simulink model "control"  (R2020a)
settings: Solver=FixedStepDiscrete  StartTime=0.0  StopTime=1  FixedStep=0.0005  RelTol=1e-3  EnableMultiTasking=on
undefined symbols (not defined in the file): acc_calmax1, acc_calmax2, acc_calmin1, acc_calmin2, akemancanshu, bre, bre_calmax, bre_calmin, ecucoder_acal, I_AN01_5K1, I_AN03_5V, I_AN04_5V, kd, ki, kp, leftmax, O_SW06_HS1A, rightmax, T_add, T_del, tiaoshi, zhiling
libraries: ec5744lib x252, canmsglib x92, simulink x5
(part 5 of 9)

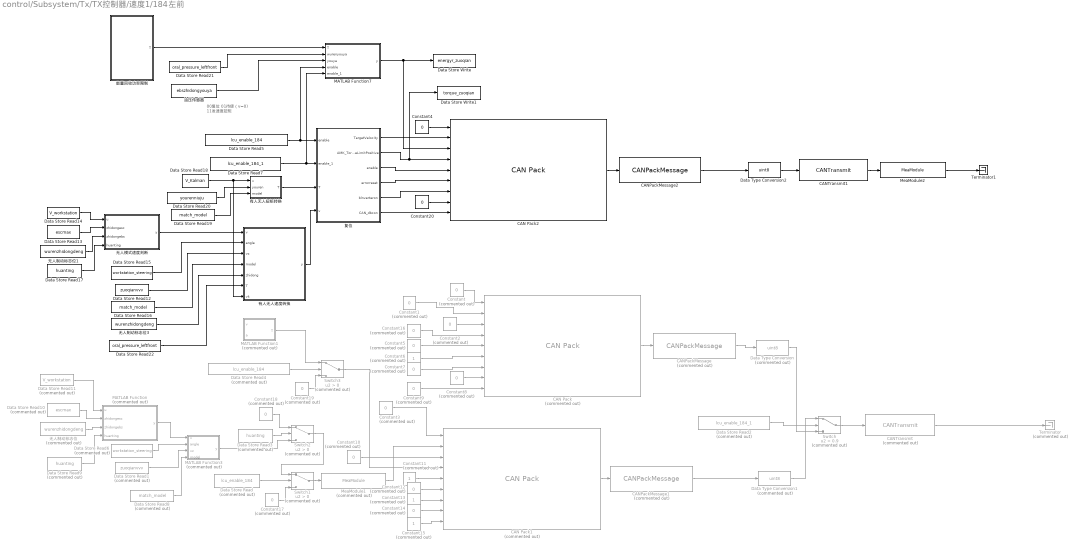
== system control/Subsystem/Tx/TX控制器/速度1/184左前 ==
  note: 00复位
      | 01待使（v=0)
      | 11发速度扭矩
  CAN Pack : canmsglib/CAN Pack  Commented=on  CANdbFile=D:\desktop\CANdbc\enable.dbc  MsgList=(none)  MsgName=first_enable  MsgIDType=Standard (11-bit identifier)  MsgIdentifier=388  MsgLength=8  Remote=off  ApplyMinMax=off  BusOutput=off  SignalInfo={'AMK_Reserve','12','4','LE','signed','Standard','0','1','0','0','15';'AMK_TargetVelocity','16','16','LE','signed','Standard','0','1','0','0','65535';'AMK_TorqueLimitNegativ','48','16','LE','signed','Standard','0','1','0','0','65535';'AMK_TorqueLimitPositiv','32','16','LE','signed','Standard','0','1','0','0','65535';'AMK_bEnable','10','1','LE','unsigned','Standard','0','1','0','0','1';'AMK_bErrorReset','11','1','LE','unsigned','Standard','0','1','0','0','1';'AMK_bInverterOn','8','1','LE','unsigned','Standard','0','1','0','0','1';'AMK_bReserve','0','8','LE','unsigned','Standard','0','1','0','0','255';'CAN_bdcon','9','1','LE','unsigned','Standard','0','1','0','0','1'}
      settings: SourceProductBaseCode=ME,XP,VN  DataFormat=CANdb specified signals
  CAN Pack1 : canmsglib/CAN Pack  Commented=on  CANdbFile=D:\desktop\CANdbc\enable.dbc  MsgList=(none)  MsgName=first_enable  MsgIDType=Standard (11-bit identifier)  MsgIdentifier=388  MsgLength=8  Remote=off  ApplyMinMax=off  BusOutput=off  SignalInfo={'AMK_Reserve','12','4','LE','signed','Standard','0','1','0','0','15';'AMK_TargetVelocity','16','16','LE','signed','Standard','0','1','0','0','65535';'AMK_TorqueLimitNegativ','48','16','LE','signed','Standard','0','1','0','0','65535';'AMK_TorqueLimitPositiv','32','16','LE','signed','Standard','0','1','0','0','65535';'AMK_bEnable','10','1','LE','unsigned','Standard','0','1','0','0','1';'AMK_bErrorReset','11','1','LE','unsigned','Standard','0','1','0','0','1';'AMK_bInverterOn','8','1','LE','unsigned','Standard','0','1','0','0','1';'AMK_bReserve','0','8','LE','unsigned','Standard','0','1','0','0','255';'CAN_bdcon','9','1','LE','unsigned','Standard','0','1','0','0','1'}
      settings: SourceProductBaseCode=ME,XP,VN  DataFormat=CANdb specified signals
  CAN Pack2 : canmsglib/CAN Pack  CANdbFile=C:\Users\86155\Desktop\HRT2024\qkx\can\enable.dbc  MsgList=first_enable  MsgName=first_enable  MsgIDType=Standard (11-bit identifier)  MsgIdentifier=388  MsgLength=8  Remote=off  ApplyMinMax=off  BusOutput=off  SignalInfo={'AMK_Reserve','12','4','LE','signed','Standard','0','1','0','-8','7';'AMK_TargetVelocity','16','16','LE','signed','Standard','0','1','0','-32768','32767';'AMK_TorqueLimitNegativ','48','16','LE','signed','Standard','0','1','0','-32768','32767';'AMK_TorqueLimitPositiv','32','16','LE','signed','Standard','0','1','0','-32768','32767';'AMK_bEnable','10','1','LE','unsigned','Standard','0','1','0','0','1';'AMK_bErrorReset','11','1','LE','unsigned','Standard','0','1','0','0','1';'AMK_bInverterOn','8','1','LE','unsigned','Standard','0','1','0','0','1';'AMK_bReserve','0','8','LE','unsigned','Standard','0','1','0','0','255';'CAN_bdcon','9','1','LE','unsigned','Standard','0','1','0','0','1'}
      settings: SourceProductBaseCode=ME,XP,VN  DataFormat=CANdb specified signals
  CANPackMessage : ec5744lib/RapidECU_U4B/04CANCommunication/CANPackMessage  Commented=on  datalength=8  sampletime=-1
      settings: SourceProductName=ECUCoder for MPC5744
  CANPackMessage1 : ec5744lib/RapidECU_U4B/04CANCommunication/CANPackMessage  Commented=on  datalength=8  sampletime=-1
      settings: SourceProductName=ECUCoder for MPC5744
  CANPackMessage2 : ec5744lib/RapidECU_U4B/04CANCommunication/CANPackMessage  datalength=8  sampletime=-1
      settings: SourceProductName=ECUCoder for MPC5744
  CANTransmit : ec5744lib/RapidECU_U4B/04CANCommunication/CANTransmit  Commented=on  canmodule=0  canbuffer=8  canmessageid=hex2dec('184')  canmessagetype=Standard(11-bit ID)  datalength=8  sampletime=-1
      settings: SourceProductName=ECUCoder for MPC5744
  CANTransmit1 : ec5744lib/RapidECU_U4B/04CANCommunication/CANTransmit  canmodule=0  canbuffer=8  canmessageid=hex2dec('184')  canmessagetype=Standard(11-bit ID)  datalength=8  sampletime=-1
      settings: SourceProductName=ECUCoder for MPC5744
  Constant{,1..3,5,7..10,12,14,16..17,19} (14 alike) : Constant  Commented=on  Value=0  SampleTime=-1
  Constant{6,11,13,15} (4 alike) : Constant  Commented=on  SampleTime=-1
  Constant18 : Constant  Commented=on  Value=0
  Constant20 : Constant  Value=0  SampleTime=-1
  Constant4 : Constant  Value=0  SampleTime=-1
  Data Store Read : DataStoreRead  Commented=on  DataStoreName=lcu_enable_184
  Data Store Read1 : DataStoreRead  Commented=on  DataStoreName=zuoqianvvv
  Data Store Read10 : DataStoreRead  Commented=on  DataStoreName=escmax
  Data Store Read11 : DataStoreRead  Commented=on  DataStoreName=V_workstation
  Data Store Read12 : DataStoreRead  DataStoreName=zuoqianvvv
  Data Store Read13 : DataStoreRead  DataStoreName=escmax
  Data Store Read14 : DataStoreRead  DataStoreName=V_workstation
  Data Store Read15 : DataStoreRead  DataStoreName=workstation_steering
  Data Store Read16 : DataStoreRead  DataStoreName=match_model
  Data Store Read17 : DataStoreRead  DataStoreName=huanting
  Data Store Read18 : DataStoreRead  DataStoreName=V_Kalman
  Data Store Read19 : DataStoreRead  DataStoreName=match_model
  Data Store Read2 : DataStoreRead  Commented=on  DataStoreName=lcu_enable_184_1
  Data Store Read20 : DataStoreRead  DataStoreName=yourenniuju
  Data Store Read21 : DataStoreRead  DataStoreName=oral_pressure_leftfront
  Data Store Read22 : DataStoreRead  DataStoreName=oral_pressure_leftfront
  Data Store Read3 : DataStoreRead  Commented=on  DataStoreName=huanting
  Data Store Read4 : DataStoreRead  Commented=on  DataStoreName=lcu_enable_184
  Data Store Read5 : DataStoreRead  DataStoreName=lcu_enable_184
  Data Store Read6 : DataStoreRead  Commented=on  DataStoreName=workstation_steering
  Data Store Read7 : DataStoreRead  DataStoreName=lcu_enable_184_1
  Data Store Read8 : DataStoreRead  Commented=on  DataStoreName=match_model
  Data Store Read9 : DataStoreRead  Commented=on  DataStoreName=huanting
  Data Store Write : DataStoreWrite  DataStoreName=energyr_zuoqian
  Data Store Write1 : DataStoreWrite  DataStoreName=torque_zuoqian
  Data Type Conversion : DataTypeConversion  Commented=on  OutDataTypeStr=uint8
  Data Type Conversion1 : DataTypeConversion  Commented=on  OutDataTypeStr=uint8
  Data Type Conversion2 : DataTypeConversion  OutDataTypeStr=uint8
  MATLAB Function : MATLAB Function  Commented=on  TreatAsAtomicUnit=on
  MATLAB Function1 : MATLAB Function  Commented=on  TreatAsAtomicUnit=on
  MATLAB Function3 : MATLAB Function  Commented=on  TreatAsAtomicUnit=on
  MATLAB Function7 : MATLAB Function  TreatAsAtomicUnit=on
  MeaModule1 : ec5744lib/RapidECU_U4B/07Calibration/MeaModule  Commented=on  signal=Vfirst
      settings: SourceProductName=ECUCoder for MPC5744
  MeaModule2 : ec5744lib/RapidECU_U4B/07Calibration/MeaModule  signal=V184
      settings: SourceProductName=ECUCoder for MPC5744
  Switch : Switch  Commented=on  Criteria=u2 > Threshold  Threshold=0.9
  Switch1 : Switch  Commented=on  Criteria=u2 > Threshold
  Switch2 : Switch  Commented=on  Criteria=u2 > Threshold
  Switch3 : Switch  Commented=on  Criteria=u2 > Threshold
  Terminator : Terminator  Commented=on
  Terminator1 : Terminator
  复位 : MATLAB Function  TreatAsAtomicUnit=on
  无人制动标志位 : DataStoreRead  Commented=on  DataStoreName=wurenzhidongdeng
  无人制动标志位1 : DataStoreRead  DataStoreName=wurenzhidongdeng
  无人制动标志位3 : DataStoreRead  DataStoreName=wurenzhidongdeng
  无人模式速度判断 : MATLAB Function  TreatAsAtomicUnit=on
  有人无人扭矩转换 : MATLAB Function  TreatAsAtomicUnit=on
  有人无人速度转换 : MATLAB Function  TreatAsAtomicUnit=on
  油压传感器 : DataStoreRead  DataStoreName=ebszhidongyouya
  能量回收功率限制 : Subsystem
  wires:
  有人无人扭矩转换/1(T) -> 复位/3(T)
  有人无人速度转换/1(y) -> 复位/4(v)
  Data Store Read13/1 -> 无人模式速度判断/2(zhidongesc)
  Data Store Read16/1 -> 有人无人速度转换/4(model)
  Data Store Read15/1 -> 有人无人速度转换/2(angle)
  Data Store Read14/1 -> 无人模式速度判断/1(u)
  无人制动标志位1/1 -> 无人模式速度判断/3(zhidongebs)
  无人模式速度判断/1(y) -> 有人无人速度转换/1(v)
  Data Store Read12/1 -> 有人无人速度转换/3(vz)
  Data Store Read17/1 -> 无人模式速度判断/4(huanting)
  Data Store Read9/1 -> MATLAB Function/4(huanting)
  Data Store Read7/1 -> MATLAB Function7/5(enable_1), 复位/2(enable_1)
  Data Store Read5/1 -> MATLAB Function7/4(enable), 复位/1("enable ")
  复位/2(AMK_TorqueLimitPositive) -> CAN Pack2/4, Data Store Write1/1
  MATLAB Function7/1(y) -> CAN Pack2/3, Data Store Write/1
  复位/6(CAN_dbcon) -> CAN Pack2/9
  复位/5(blnverteron) -> CAN Pack2/7
  复位/4(errorreset) -> CAN Pack2/6
  复位/3(enable) -> CAN Pack2/5
  复位/1(TargetVelocity) -> CAN Pack2/2
  Constant20/1 -> CAN Pack2/8
  Constant4/1 -> CAN Pack2/1
  Data Type Conversion2/1 -> CANTransmit1/1
  CANTransmit1/1 -> MeaModule2/1
  CANPackMessage2/1 -> Data Type Conversion2/1
  CAN Pack2/1 -> CANPackMessage2/1
  MeaModule2/1 -> Terminator1/1
  Data Store Read1/1 -> MATLAB Function3/3(vz)
  Data Store Read11/1 -> MATLAB Function/1(u)
  无人制动标志位/1 -> MATLAB Function/3(zhidongebs)
  Data Store Read10/1 -> MATLAB Function/2(zhidongesc)
  Data Store Read8/1 -> MATLAB Function3/4(model)
  Data Store Read6/1 -> MATLAB Function3/2(angle)
  MATLAB Function3/1(y) -> Switch2/3
  MATLAB Function/1(y) -> MATLAB Function3/1(v)
  MATLAB Function1/1(T) -> Switch3/1
  Switch3/1 -> CAN Pack1/4
  Constant19/1 -> Switch3/3
  Data Store Read4/1 -> Switch3/2
  MeaModule1/1 -> CAN Pack1/2
  Switch2/1 -> Switch1/1
  Constant18/1 -> Switch2/1
  Data Store Read3/1 -> Switch2/2
  Data Store Read2/1 -> Switch/2
  Constant17/1 -> Switch1/3
  Data Store Read/1 -> Switch1/2
  Switch1/1 -> MeaModule1/1
  Data Type Conversion/1 -> Switch/3
  CANPackMessage/1 -> Data Type Conversion/1
  Switch/1 -> CANTransmit/1
  Constant10/1 -> CAN Pack1/3
  Data Type Conversion1/1 -> Switch/1
  Constant11/1 -> CAN Pack1/5
  Constant15/1 -> CAN Pack1/9
  CANPackMessage1/1 -> Data Type Conversion1/1
  Constant12/1 -> CAN Pack1/6
  CAN Pack1/1 -> CANPackMessage1/1
  Constant13/1 -> CAN Pack1/7
  Constant3/1 -> CAN Pack1/1
  Constant14/1 -> CAN Pack1/8
  CANTransmit/1 -> Terminator/1
  Constant6/1 -> CAN Pack/6
  Constant2/1 -> CAN Pack/3
  Constant16/1 -> CAN Pack/4
  Constant1/1 -> CAN Pack/2
  Constant7/1 -> CAN Pack/7
  CAN Pack/1 -> CANPackMessage/1
  Constant9/1 -> CAN Pack/9
  Constant/1 -> CAN Pack/1
  Constant5/1 -> CAN Pack/5
  Constant8/1 -> CAN Pack/8
  Data Store Read18/1 -> 有人无人速度转换/7(vk), 有人无人扭矩转换/1(v)
  Data Store Read19/1 -> 有人无人扭矩转换/3(model)
  Data Store Read20/1 -> 有人无人扭矩转换/2(youren)
  油压传感器/1 -> MATLAB Function7/3(youya)
  Data Store Read21/1 -> MATLAB Function7/2(wurenyouya)
  无人制动标志位3/1 -> 有人无人速度转换/5(zhidong)
  能量回收功率限制/1(T) -> MATLAB Function7/1(T)
  Data Store Read22/1 -> 有人无人速度转换/6(T)

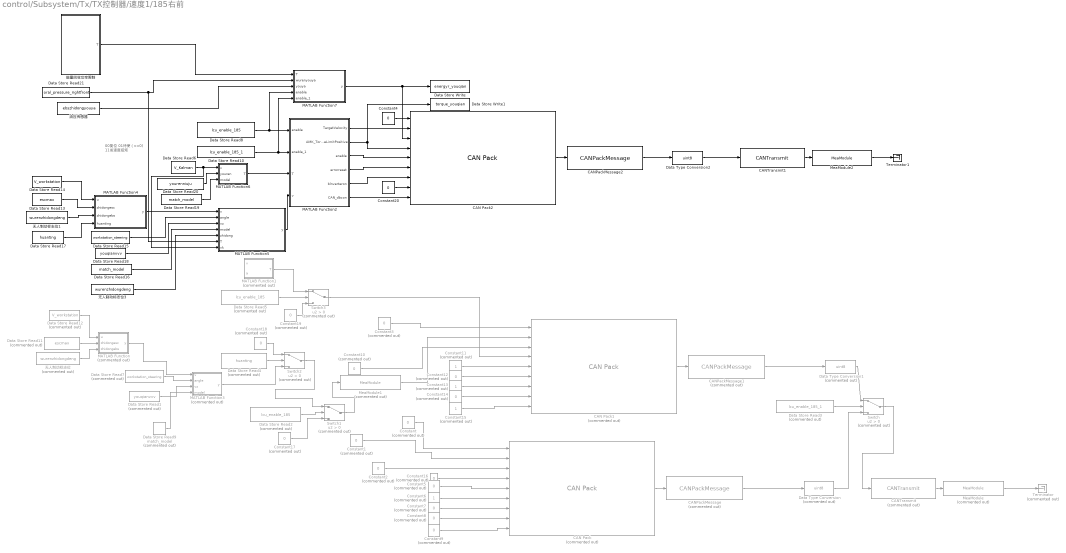
== system control/Subsystem/Tx/TX控制器/速度1/185右前 ==
  note: 00复位
      | 01待使（v=0)
      | 11发速度扭矩
  CAN Pack : canmsglib/CAN Pack  Commented=on  CANdbFile=D:\desktop\CANdbc\enable - youqian.dbc  MsgList=(none)  MsgName=first_enable  MsgIDType=Standard (11-bit identifier)  MsgIdentifier=389  MsgLength=8  Remote=off  ApplyMinMax=off  BusOutput=off  SignalInfo={'AMK_Reserve','12','4','LE','signed','Standard','0','1','0','0','15';'AMK_TargetVelocity','16','16','LE','signed','Standard','0','1','0','0','65535';'AMK_TorqueLimitNegativ','48','16','LE','signed','Standard','0','1','0','0','65535';'AMK_TorqueLimitPositiv','32','16','LE','signed','Standard','0','1','0','0','65535';'AMK_bEnable','10','1','LE','unsigned','Standard','0','1','0','0','1';'AMK_bErrorReset','11','1','LE','unsigned','Standard','0','1','0','0','1';'AMK_bInverterOn','8','1','LE','unsigned','Standard','0','1','0','0','1';'AMK_bReserve','0','8','LE','unsigned','Standard','0','1','0','0','255';'CAN_bdcon','9','1','LE','unsigned','Standard','0','1','0','0','1'}
      settings: SourceProductBaseCode=ME,XP,VN  DataFormat=CANdb specified signals
  CAN Pack1 : canmsglib/CAN Pack  Commented=on  CANdbFile=D:\desktop\CANdbc\enable - youqian.dbc  MsgList=(none)  MsgName=first_enable  MsgIDType=Standard (11-bit identifier)  MsgIdentifier=389  MsgLength=8  Remote=off  ApplyMinMax=off  BusOutput=off  SignalInfo={'AMK_Reserve','12','4','LE','signed','Standard','0','1','0','0','15';'AMK_TargetVelocity','16','16','LE','signed','Standard','0','1','0','0','65535';'AMK_TorqueLimitNegativ','48','16','LE','signed','Standard','0','1','0','0','65535';'AMK_TorqueLimitPositiv','32','16','LE','signed','Standard','0','1','0','0','65535';'AMK_bEnable','10','1','LE','unsigned','Standard','0','1','0','0','1';'AMK_bErrorReset','11','1','LE','unsigned','Standard','0','1','0','0','1';'AMK_bInverterOn','8','1','LE','unsigned','Standard','0','1','0','0','1';'AMK_bReserve','0','8','LE','unsigned','Standard','0','1','0','0','255';'CAN_bdcon','9','1','LE','unsigned','Standard','0','1','0','0','1'}
      settings: SourceProductBaseCode=ME,XP,VN  DataFormat=CANdb specified signals
  CAN Pack2 : canmsglib/CAN Pack  CANdbFile=C:\Users\86155\Desktop\HRT2024\qkx\can\enable.dbc  MsgList=first_enable  MsgName=first_enable  MsgIDType=Standard (11-bit identifier)  MsgIdentifier=388  MsgLength=8  Remote=off  ApplyMinMax=off  BusOutput=off  SignalInfo={'AMK_Reserve','12','4','LE','signed','Standard','0','1','0','-8','7';'AMK_TargetVelocity','16','16','LE','signed','Standard','0','1','0','-32768','32767';'AMK_TorqueLimitNegativ','48','16','LE','signed','Standard','0','1','0','-32768','32767';'AMK_TorqueLimitPositiv','32','16','LE','signed','Standard','0','1','0','-32768','32767';'AMK_bEnable','10','1','LE','unsigned','Standard','0','1','0','0','1';'AMK_bErrorReset','11','1','LE','unsigned','Standard','0','1','0','0','1';'AMK_bInverterOn','8','1','LE','unsigned','Standard','0','1','0','0','1';'AMK_bReserve','0','8','LE','unsigned','Standard','0','1','0','0','255';'CAN_bdcon','9','1','LE','unsigned','Standard','0','1','0','0','1'}
      settings: SourceProductBaseCode=ME,XP,VN  DataFormat=CANdb specified signals
  CANPackMessage : ec5744lib/RapidECU_U4B/04CANCommunication/CANPackMessage  Commented=on  datalength=8  sampletime=-1
      settings: SourceProductName=ECUCoder for MPC5744
  CANPackMessage1 : ec5744lib/RapidECU_U4B/04CANCommunication/CANPackMessage  Commented=on  datalength=8  sampletime=-1
      settings: SourceProductName=ECUCoder for MPC5744
  CANPackMessage2 : ec5744lib/RapidECU_U4B/04CANCommunication/CANPackMessage  datalength=8  sampletime=-1
      settings: SourceProductName=ECUCoder for MPC5744
  CANTransmit : ec5744lib/RapidECU_U4B/04CANCommunication/CANTransmit  Commented=on  canmodule=0  canbuffer=11  canmessageid=hex2dec('185')  canmessagetype=Standard(11-bit ID)  datalength=8  sampletime=-1
      settings: SourceProductName=ECUCoder for MPC5744
  CANTransmit1 : ec5744lib/RapidECU_U4B/04CANCommunication/CANTransmit  canmodule=0  canbuffer=11  canmessageid=hex2dec('185')  canmessagetype=Standard(11-bit ID)  datalength=8  sampletime=-1
      settings: SourceProductName=ECUCoder for MPC5744
  Constant{,1..3,5,7..10,12,14,16..17,19} (14 alike) : Constant  Commented=on  Value=0  SampleTime=-1
  Constant{6,11,13,15} (4 alike) : Constant  Commented=on  SampleTime=-1
  Constant18 : Constant  Commented=on  Value=0
  Constant20 : Constant  Value=0  SampleTime=-1
  Constant4 : Constant  Value=0  SampleTime=-1
  Data Store Read1 : DataStoreRead  Commented=on  DataStoreName=youqianvvv
  Data Store Read10 : DataStoreRead  DataStoreName=lcu_enable_185_1
  Data Store Read11 : DataStoreRead  Commented=on  DataStoreName=escmax
  Data Store Read12 : DataStoreRead  Commented=on  DataStoreName=V_workstation
  Data Store Read13 : DataStoreRead  DataStoreName=escmax
  Data Store Read14 : DataStoreRead  DataStoreName=V_workstation
  Data Store Read15 : DataStoreRead  DataStoreName=workstation_steering
  Data Store Read16 : DataStoreRead  DataStoreName=match_model
  Data Store Read17 : DataStoreRead  DataStoreName=huanting
  Data Store Read18 : DataStoreRead  DataStoreName=youqianvvv
  Data Store Read19 : DataStoreRead  DataStoreName=match_model
  Data Store Read2 : DataStoreRead  Commented=on  DataStoreName=lcu_enable_185
  Data Store Read20 : DataStoreRead  DataStoreName=yourenniuju
  Data Store Read21 : DataStoreRead  DataStoreName=oral_pressure_rightfront
  Data Store Read3 : DataStoreRead  Commented=on  DataStoreName=lcu_enable_185_1
  Data Store Read4 : DataStoreRead  Commented=on  DataStoreName=huanting
  Data Store Read5 : DataStoreRead  Commented=on  DataStoreName=lcu_enable_185
  Data Store Read6 : DataStoreRead  DataStoreName=V_Kalman
  Data Store Read7 : DataStoreRead  Commented=on  DataStoreName=workstation_steering
  Data Store Read8 : DataStoreRead  DataStoreName=lcu_enable_185
  Data Store Read9 : DataStoreRead  Commented=on  DataStoreName=match_model
  Data Store Write : DataStoreWrite  DataStoreName=energyr_youqian
  Data Store Write1 : DataStoreWrite  DataStoreName=torque_youqian
  Data Type Conversion : DataTypeConversion  Commented=on  OutDataTypeStr=uint8
  Data Type Conversion1 : DataTypeConversion  Commented=on  OutDataTypeStr=uint8
  Data Type Conversion2 : DataTypeConversion  OutDataTypeStr=uint8
  MATLAB Function : MATLAB Function  Commented=on  TreatAsAtomicUnit=on
  MATLAB Function1 : MATLAB Function  Commented=on  TreatAsAtomicUnit=on
  MATLAB Function2 : MATLAB Function  TreatAsAtomicUnit=on
  MATLAB Function3 : MATLAB Function  Commented=on  TreatAsAtomicUnit=on
  MATLAB Function4 : MATLAB Function  TreatAsAtomicUnit=on
  MATLAB Function5 : MATLAB Function  TreatAsAtomicUnit=on
  MATLAB Function6 : MATLAB Function  TreatAsAtomicUnit=on
  MATLAB Function7 : MATLAB Function  TreatAsAtomicUnit=on
  MeaModule : ec5744lib/RapidECU_U4B/07Calibration/MeaModule  Commented=on  signal=V185
      settings: SourceProductName=ECUCoder for MPC5744
  MeaModule1 : ec5744lib/RapidECU_U4B/07Calibration/MeaModule  Commented=on  signal=Vforth
      settings: SourceProductName=ECUCoder for MPC5744
  MeaModule2 : ec5744lib/RapidECU_U4B/07Calibration/MeaModule  signal=V185
      settings: SourceProductName=ECUCoder for MPC5744
  Switch{,1..3} (4 alike) : Switch  Commented=on  Criteria=u2 > Threshold
  Terminator : Terminator  Commented=on
  Terminator1 : Terminator
  无人制动标志位 : DataStoreRead  Commented=on  DataStoreName=wurenzhidongdeng
  无人制动标志位1 : DataStoreRead  DataStoreName=wurenzhidongdeng
  无人制动标志位3 : DataStoreRead  DataStoreName=wurenzhidongdeng
  油压传感器 : DataStoreRead  DataStoreName=ebszhidongyouya
  能量回收功率限制 : Subsystem
  wires:
  Data Store Read10/1 -> MATLAB Function7/5(enable_1), MATLAB Function2/2(enable_1)
  Data Type Conversion2/1 -> CANTransmit1/1
  CAN Pack2/1 -> CANPackMessage2/1
  MeaModule2/1 -> Terminator1/1
  CANTransmit1/1 -> MeaModule2/1
  CANPackMessage2/1 -> Data Type Conversion2/1
  Data Store Read17/1 -> MATLAB Function4/4(huanting)
  MATLAB Function5/1(y) -> MATLAB Function2/4(v)
  无人制动标志位1/1 -> MATLAB Function4/3(zhidongebs)
  Data Store Read14/1 -> MATLAB Function4/1(u)
  Data Store Read15/1 -> MATLAB Function5/2(angle)
  Data Store Read13/1 -> MATLAB Function4/2(zhidongesc)
  Data Store Read16/1 -> MATLAB Function5/4(model)
  MATLAB Function6/1(T) -> MATLAB Function2/3(T)
  Data Store Read8/1 -> MATLAB Function7/4(enable), MATLAB Function2/1("enable ")
  MATLAB Function2/4(errorreset) -> CAN Pack2/6
  MATLAB Function2/1(TargetVelocity) -> CAN Pack2/2
  Constant4/1 -> CAN Pack2/1
  MATLAB Function2/2(AMK_TorqueLimitPositive) -> Data Store Write1/1, CAN Pack2/4
  MATLAB Function2/6(CAN_dbcon) -> CAN Pack2/9
  Constant20/1 -> CAN Pack2/8
  MATLAB Function2/5(blnverteron) -> CAN Pack2/7
  MATLAB Function2/3(enable) -> CAN Pack2/5
  Data Store Read18/1 -> MATLAB Function5/3(vz)
  Data Store Read12/1 -> MATLAB Function/1(u)
  Data Store Read11/1 -> MATLAB Function/2(zhidongesc)
  MATLAB Function/1(y) -> MATLAB Function3/1(v)
  无人制动标志位/1 -> MATLAB Function/3(zhidongebs)
  MATLAB Function1/1(T) -> Switch3/1
  Data Store Read9/1 -> MATLAB Function3/4(model)
  MATLAB Function3/1(y) -> Switch2/3
  Data Store Read1/1 -> MATLAB Function3/3(vz)
  Data Store Read7/1 -> MATLAB Function3/2(angle)
  Data Store Read5/1 -> Switch3/2
  Switch3/1 -> CAN Pack1/4
  Constant19/1 -> Switch3/3
  MeaModule1/1 -> CAN Pack1/2
  Switch2/1 -> Switch1/1
  Constant18/1 -> Switch2/1
  Data Store Read4/1 -> Switch2/2
  Data Store Read2/1 -> Switch1/2
  Constant17/1 -> Switch1/3
  Switch1/1 -> MeaModule1/1
  Data Store Read3/1 -> Switch/2
  Switch/1 -> CANTransmit/1
  Data Type Conversion/1 -> Switch/3
  Data Type Conversion1/1 -> Switch/1
  Constant15/1 -> CAN Pack1/9
  Constant14/1 -> CAN Pack1/8
  Constant10/1 -> CAN Pack1/3
  CAN Pack1/1 -> CANPackMessage1/1
  Constant13/1 -> CAN Pack1/7
  Constant12/1 -> CAN Pack1/6
  Constant11/1 -> CAN Pack1/5
  Constant3/1 -> CAN Pack1/1
  CANPackMessage1/1 -> Data Type Conversion1/1
  MeaModule/1 -> Terminator/1
  CANTransmit/1 -> MeaModule/1
  Constant6/1 -> CAN Pack/6
  Constant2/1 -> CAN Pack/3
  Constant16/1 -> CAN Pack/4
  Constant1/1 -> CAN Pack/2
  Constant7/1 -> CAN Pack/7
  CAN Pack/1 -> CANPackMessage/1
  Constant9/1 -> CAN Pack/9
  CANPackMessage/1 -> Data Type Conversion/1
  Constant/1 -> CAN Pack/1
  Constant5/1 -> CAN Pack/5
  Constant8/1 -> CAN Pack/8
  Data Store Read19/1 -> MATLAB Function6/3(model)
  Data Store Read20/1 -> MATLAB Function6/2(youren)
  Data Store Read6/1 -> MATLAB Function5/7(vk), MATLAB Function6/1(v)
  MATLAB Function4/1(y) -> MATLAB Function5/1(v)
  无人制动标志位3/1 -> MATLAB Function5/5(zhidong)
  能量回收功率限制/1(T) -> MATLAB Function7/1(T)
  油压传感器/1 -> MATLAB Function7/3(youya)
  Data Store Read21/1 -> MATLAB Function5/6(T), MATLAB Function7/2(wurenyouya)
  MATLAB Function7/1(y) -> CAN Pack2/3, Data Store Write/1

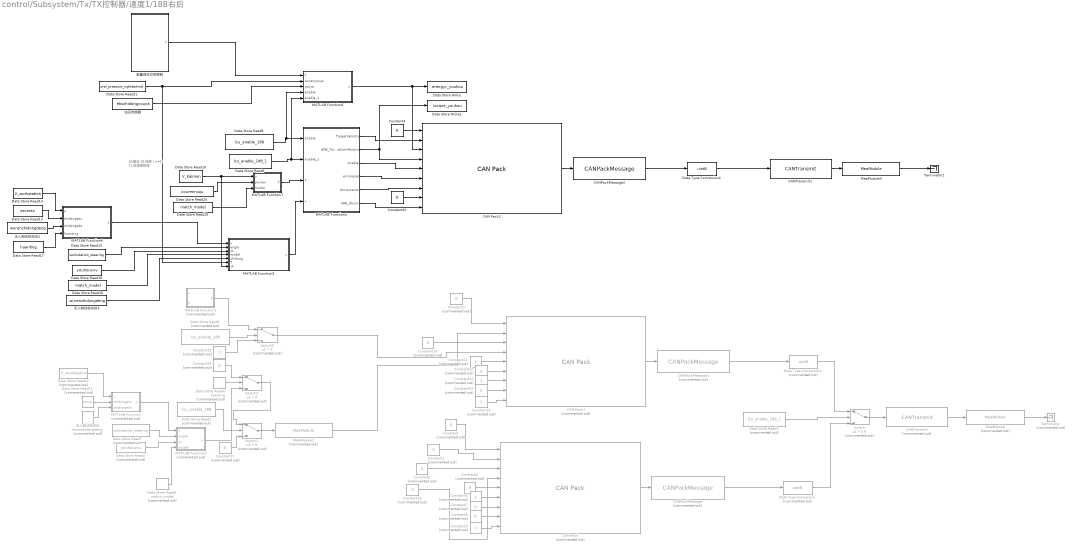
== system control/Subsystem/Tx/TX控制器/速度1/188右后 ==
  note: 00复位
      | 01待使（v=0)
      | 11发速度扭矩
  CAN Pack : canmsglib/CAN Pack  Commented=on  CANdbFile=D:\desktop\CANdbc\enable - zuohou - 副本.dbc  MsgList=(none)  MsgName=first_enable  MsgIDType=Standard (11-bit identifier)  MsgIdentifier=392  MsgLength=8  Remote=off  ApplyMinMax=off  BusOutput=off  SignalInfo={'AMK_Reserve','12','4','LE','signed','Standard','0','1','0','0','15';'AMK_TargetVelocity','16','16','LE','signed','Standard','0','1','0','0','65535';'AMK_TorqueLimitNegativ','48','16','LE','signed','Standard','0','1','0','0','65535';'AMK_TorqueLimitPositiv','32','16','LE','signed','Standard','0','1','0','0','65535';'AMK_bEnable','10','1','LE','unsigned','Standard','0','1','0','0','1';'AMK_bErrorReset','11','1','LE','unsigned','Standard','0','1','0','0','1';'AMK_bInverterOn','8','1','LE','unsigned','Standard','0','1','0','0','1';'AMK_bReserve','0','8','LE','unsigned','Standard','0','1','0','0','255';'CAN_bdcon','9','1','LE','unsigned','Standard','0','1','0','0','1'}
      settings: SourceProductBaseCode=ME,XP,VN  DataFormat=CANdb specified signals
  CAN Pack1 : canmsglib/CAN Pack  Commented=on  CANdbFile=D:\desktop\CANdbc\enable - zuohou - 副本.dbc  MsgList=(none)  MsgName=first_enable  MsgIDType=Standard (11-bit identifier)  MsgIdentifier=392  MsgLength=8  Remote=off  ApplyMinMax=off  BusOutput=off  SignalInfo={'AMK_Reserve','12','4','LE','signed','Standard','0','1','0','0','15';'AMK_TargetVelocity','16','16','LE','signed','Standard','0','1','0','0','65535';'AMK_TorqueLimitNegativ','48','16','LE','signed','Standard','0','1','0','0','65535';'AMK_TorqueLimitPositiv','32','16','LE','signed','Standard','0','1','0','0','65535';'AMK_bEnable','10','1','LE','unsigned','Standard','0','1','0','0','1';'AMK_bErrorReset','11','1','LE','unsigned','Standard','0','1','0','0','1';'AMK_bInverterOn','8','1','LE','unsigned','Standard','0','1','0','0','1';'AMK_bReserve','0','8','LE','unsigned','Standard','0','1','0','0','255';'CAN_bdcon','9','1','LE','unsigned','Standard','0','1','0','0','1'}
      settings: SourceProductBaseCode=ME,XP,VN  DataFormat=CANdb specified signals
  CAN Pack2 : canmsglib/CAN Pack  CANdbFile=C:\Users\86155\Desktop\HRT2024\qkx\can\enable.dbc  MsgList=first_enable  MsgName=first_enable  MsgIDType=Standard (11-bit identifier)  MsgIdentifier=388  MsgLength=8  Remote=off  ApplyMinMax=off  BusOutput=off  SignalInfo={'AMK_Reserve','12','4','LE','signed','Standard','0','1','0','-8','7';'AMK_TargetVelocity','16','16','LE','signed','Standard','0','1','0','-32768','32767';'AMK_TorqueLimitNegativ','48','16','LE','signed','Standard','0','1','0','-32768','32767';'AMK_TorqueLimitPositiv','32','16','LE','signed','Standard','0','1','0','-32768','32767';'AMK_bEnable','10','1','LE','unsigned','Standard','0','1','0','0','1';'AMK_bErrorReset','11','1','LE','unsigned','Standard','0','1','0','0','1';'AMK_bInverterOn','8','1','LE','unsigned','Standard','0','1','0','0','1';'AMK_bReserve','0','8','LE','unsigned','Standard','0','1','0','0','255';'CAN_bdcon','9','1','LE','unsigned','Standard','0','1','0','0','1'}
      settings: SourceProductBaseCode=ME,XP,VN  DataFormat=CANdb specified signals
  CANPackMessage : ec5744lib/RapidECU_U4B/04CANCommunication/CANPackMessage  Commented=on  datalength=8  sampletime=-1
      settings: SourceProductName=ECUCoder for MPC5744
  CANPackMessage1 : ec5744lib/RapidECU_U4B/04CANCommunication/CANPackMessage  Commented=on  datalength=8  sampletime=-1
      settings: SourceProductName=ECUCoder for MPC5744
  CANPackMessage2 : ec5744lib/RapidECU_U4B/04CANCommunication/CANPackMessage  datalength=8  sampletime=-1
      settings: SourceProductName=ECUCoder for MPC5744
  CANTransmit : ec5744lib/RapidECU_U4B/04CANCommunication/CANTransmit  Commented=on  canmodule=0  canbuffer=9  canmessageid=hex2dec('188')  canmessagetype=Standard(11-bit ID)  datalength=8  sampletime=-1
      settings: SourceProductName=ECUCoder for MPC5744
  CANTransmit1 : ec5744lib/RapidECU_U4B/04CANCommunication/CANTransmit  canmodule=0  canbuffer=9  canmessageid=hex2dec('188')  canmessagetype=Standard(11-bit ID)  datalength=8  sampletime=-1
      settings: SourceProductName=ECUCoder for MPC5744
  Constant{,1..3,5,7..10,12,14,17,19} (13 alike) : Constant  Commented=on  Value=0  SampleTime=-1
  Constant{6,11,13,15} (4 alike) : Constant  Commented=on  SampleTime=-1
  Constant16 : Constant  Commented=on  Value=0
  Constant18 : Constant  Commented=on  Value=0
  Constant20 : Constant  Value=0  SampleTime=-1
  Constant4 : Constant  Value=0  SampleTime=-1
  Data Store Read1 : DataStoreRead  Commented=on  DataStoreName=lcu_enable_188
  Data Store Read10 : DataStoreRead  DataStoreName=V_Kalman
  Data Store Read11 : DataStoreRead  Commented=on  DataStoreName=escmax
  Data Store Read12 : DataStoreRead  Commented=on  DataStoreName=V_workstation
  Data Store Read13 : DataStoreRead  DataStoreName=escmax
  Data Store Read14 : DataStoreRead  DataStoreName=V_workstation
  Data Store Read15 : DataStoreRead  DataStoreName=workstation_steering
  Data Store Read16 : DataStoreRead  DataStoreName=match_model
  Data Store Read17 : DataStoreRead  DataStoreName=huanting
  Data Store Read18 : DataStoreRead  DataStoreName=youhouvvv
  Data Store Read19 : DataStoreRead  DataStoreName=match_model
  Data Store Read2 : DataStoreRead  Commented=on  DataStoreName=youhouvvv
  Data Store Read20 : DataStoreRead  DataStoreName=yourenniuju
  Data Store Read21 : DataStoreRead  DataStoreName=oral_pressure_rightbehind
  Data Store Read3 : DataStoreRead  Commented=on  DataStoreName=lcu_enable_188_1
  Data Store Read4 : DataStoreRead  Commented=on  DataStoreName=huanting
  Data Store Read5 : DataStoreRead  Commented=on  DataStoreName=lcu_enable_188
  Data Store Read6 : DataStoreRead  DataStoreName=lcu_enable_188_1
  Data Store Read7 : DataStoreRead  Commented=on  DataStoreName=workstation_steering
  Data Store Read8 : DataStoreRead  DataStoreName=lcu_enable_188
  Data Store Read9 : DataStoreRead  Commented=on  DataStoreName=match_model
  Data Store Write : DataStoreWrite  DataStoreName=energyr_youhou
  Data Store Write1 : DataStoreWrite  DataStoreName=torque_youhou
  Data Type Conversion : DataTypeConversion  Commented=on  OutDataTypeStr=uint8
  Data Type Conversion1 : DataTypeConversion  Commented=on  OutDataTypeStr=uint8
  Data Type Conversion2 : DataTypeConversion  OutDataTypeStr=uint8
  MATLAB Function : MATLAB Function  Commented=on  TreatAsAtomicUnit=on
  MATLAB Function1 : MATLAB Function  Commented=on  TreatAsAtomicUnit=on
  MATLAB Function2 : MATLAB Function  TreatAsAtomicUnit=on
  MATLAB Function3 : MATLAB Function  Commented=on  TreatAsAtomicUnit=on
  MATLAB Function4 : MATLAB Function  TreatAsAtomicUnit=on
  MATLAB Function5 : MATLAB Function  TreatAsAtomicUnit=on
  MATLAB Function6 : MATLAB Function  TreatAsAtomicUnit=on
  MATLAB Function7 : MATLAB Function  TreatAsAtomicUnit=on
  MeaModule : ec5744lib/RapidECU_U4B/07Calibration/MeaModule  Commented=on  signal=V188
      settings: SourceProductName=ECUCoder for MPC5744
  MeaModule1 : ec5744lib/RapidECU_U4B/07Calibration/MeaModule  Commented=on  signal=Vsecond
      settings: SourceProductName=ECUCoder for MPC5744
  MeaModule3 : ec5744lib/RapidECU_U4B/07Calibration/MeaModule  signal=V188
      settings: SourceProductName=ECUCoder for MPC5744
  Switch : Switch  Commented=on  Criteria=u2 > Threshold  Threshold=0.9
  Switch1 : Switch  Commented=on  Criteria=u2 > Threshold
  Switch2 : Switch  Commented=on  Criteria=u2 > Threshold
  Switch3 : Switch  Commented=on  Criteria=u2 > Threshold
  Terminator : Terminator  Commented=on
  Terminator1 : Terminator
  无人制动标志位 : DataStoreRead  Commented=on  DataStoreName=wurenzhidongdeng
  无人制动标志位1 : DataStoreRead  DataStoreName=wurenzhidongdeng
  无人制动标志位3 : DataStoreRead  DataStoreName=wurenzhidongdeng
  油压传感器 : DataStoreRead  DataStoreName=ebszhidongyouya
  能量回收功率限制 : Subsystem
  wires:
  CANPackMessage2/1 -> Data Type Conversion2/1
  CAN Pack2/1 -> CANPackMessage2/1
  CANTransmit1/1 -> MeaModule3/1
  Data Store Read16/1 -> MATLAB Function5/4(model)
  MATLAB Function2/1(TargetVelocity) -> CAN Pack2/2
  Constant20/1 -> CAN Pack2/8
  Data Type Conversion2/1 -> CANTransmit1/1
  MATLAB Function7/1(T) -> MATLAB Function2/3(T)
  MeaModule3/1 -> Terminator1/1
  MATLAB Function2/5(blnverteron) -> CAN Pack2/7
  MATLAB Function2/4(errorreset) -> CAN Pack2/6
  MATLAB Function2/3(enable) -> CAN Pack2/5
  MATLAB Function2/6(CAN_dbcon) -> CAN Pack2/9
  MATLAB Function2/2(AMK_TorqueLimitPositive) -> CAN Pack2/4, Data Store Write1/1
  Data Store Read6/1 -> MATLAB Function6/5(enable_1), MATLAB Function2/2(enable_1)
  Constant4/1 -> CAN Pack2/1
  Data Store Read8/1 -> MATLAB Function6/4(enable), MATLAB Function2/1("enable ")
  MATLAB Function5/1(y) -> MATLAB Function2/4(v)
  Data Store Read17/1 -> MATLAB Function4/4(huanting)
  Data Store Read18/1 -> MATLAB Function5/3(vz)
  Data Store Read13/1 -> MATLAB Function4/2(zhidongesc)
  MATLAB Function4/1(y) -> MATLAB Function5/1(v)
  无人制动标志位1/1 -> MATLAB Function4/3(zhidongebs)
  Data Store Read15/1 -> MATLAB Function5/2(angle)
  Data Store Read14/1 -> MATLAB Function4/1(u)
  Data Store Read2/1 -> MATLAB Function3/3(vz)
  Data Store Read12/1 -> MATLAB Function/1(u)
  Data Store Read11/1 -> MATLAB Function/2(zhidongesc)
  MATLAB Function/1(y) -> MATLAB Function3/1(v)
  无人制动标志位/1 -> MATLAB Function/3(zhidongebs)
  MATLAB Function1/1(T) -> Switch3/1
  Data Store Read9/1 -> MATLAB Function3/4(model)
  MATLAB Function3/1(y) -> Switch2/3
  Data Store Read7/1 -> MATLAB Function3/2(angle)
  Data Store Read5/1 -> Switch3/2
  Constant19/1 -> Switch3/3
  Switch3/1 -> CAN Pack1/4
  MeaModule1/1 -> CAN Pack1/2
  Switch2/1 -> Switch1/1
  Constant18/1 -> Switch2/1
  Data Store Read4/1 -> Switch2/2
  Switch1/1 -> MeaModule1/1
  Data Store Read1/1 -> Switch1/2
  Constant17/1 -> Switch1/3
  Switch/1 -> CANTransmit/1
  Data Type Conversion/1 -> Switch/3
  Data Store Read3/1 -> Switch/2
  Constant13/1 -> CAN Pack1/7
  Constant15/1 -> CAN Pack1/9
  CAN Pack1/1 -> CANPackMessage1/1
  Constant11/1 -> CAN Pack1/5
  Constant3/1 -> CAN Pack1/1
  Constant14/1 -> CAN Pack1/8
  CANPackMessage1/1 -> Data Type Conversion1/1
  Constant10/1 -> CAN Pack1/3
  Constant12/1 -> CAN Pack1/6
  Data Type Conversion1/1 -> Switch/1
  MeaModule/1 -> Terminator/1
  CANTransmit/1 -> MeaModule/1
  Constant6/1 -> CAN Pack/6
  Constant2/1 -> CAN Pack/3
  Constant16/1 -> CAN Pack/4
  Constant1/1 -> CAN Pack/2
  Constant7/1 -> CAN Pack/7
  CAN Pack/1 -> CANPackMessage/1
  Constant9/1 -> CAN Pack/9
  CANPackMessage/1 -> Data Type Conversion/1
  Constant/1 -> CAN Pack/1
  Constant5/1 -> CAN Pack/5
  Constant8/1 -> CAN Pack/8
  Data Store Read19/1 -> MATLAB Function7/3(model)
  Data Store Read20/1 -> MATLAB Function7/2(youren)
  Data Store Read10/1 -> MATLAB Function7/1(v), MATLAB Function5/7(vk)
  无人制动标志位3/1 -> MATLAB Function5/5(zhidong)
  能量回收功率限制/1(T) -> MATLAB Function6/1(T)
  油压传感器/1 -> MATLAB Function6/3(youya)
  Data Store Read21/1 -> MATLAB Function5/6(T), MATLAB Function6/2(wurenyouya)
  MATLAB Function6/1(y) -> Data Store Write/1, CAN Pack2/3

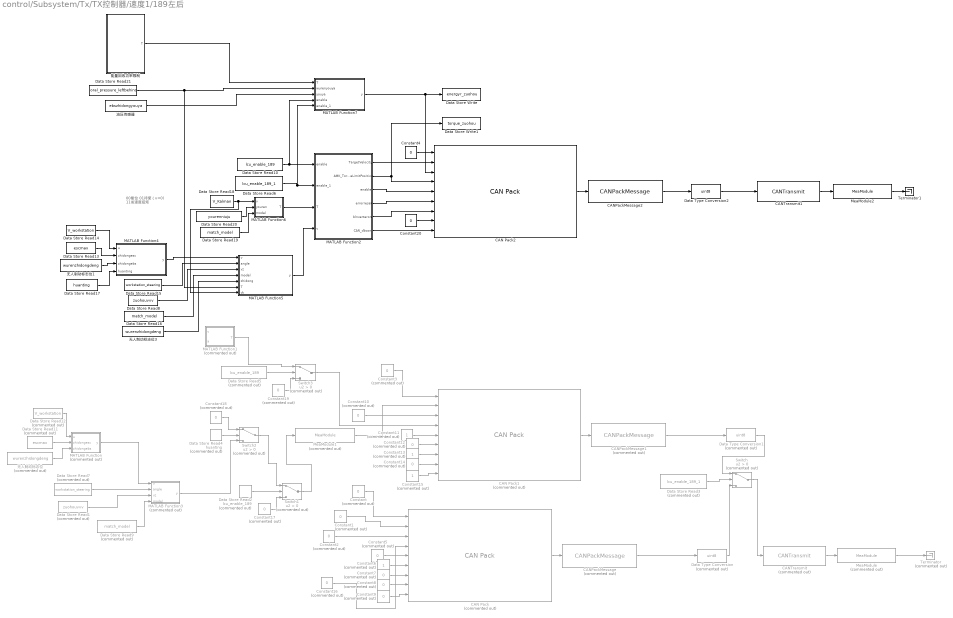
== system control/Subsystem/Tx/TX控制器/速度1/189左后 ==
  note: 00复位
      | 01待使（v=0)
      | 11发速度扭矩
  CAN Pack : canmsglib/CAN Pack  Commented=on  CANdbFile=D:\desktop\CANdbc\enable - youhou -.dbc  MsgList=(none)  MsgName=first_enable  MsgIDType=Standard (11-bit identifier)  MsgIdentifier=393  MsgLength=8  Remote=off  ApplyMinMax=off  BusOutput=off  SignalInfo={'AMK_Reserve','12','4','LE','signed','Standard','0','1','0','0','15';'AMK_TargetVelocity','16','16','LE','signed','Standard','0','1','0','0','65535';'AMK_TorqueLimitNegativ','48','16','LE','signed','Standard','0','1','0','0','65535';'AMK_TorqueLimitPositiv','32','16','LE','signed','Standard','0','1','0','0','65535';'AMK_bEnable','10','1','LE','unsigned','Standard','0','1','0','0','1';'AMK_bErrorReset','11','1','LE','unsigned','Standard','0','1','0','0','1';'AMK_bInverterOn','8','1','LE','unsigned','Standard','0','1','0','0','1';'AMK_bReserve','0','8','LE','unsigned','Standard','0','1','0','0','255';'CAN_bdcon','9','1','LE','unsigned','Standard','0','1','0','0','1'}
      settings: SourceProductBaseCode=ME,XP,VN  DataFormat=CANdb specified signals
  CAN Pack1 : canmsglib/CAN Pack  Commented=on  CANdbFile=D:\desktop\CANdbc\enable - youhou -.dbc  MsgList=(none)  MsgName=first_enable  MsgIDType=Standard (11-bit identifier)  MsgIdentifier=393  MsgLength=8  Remote=off  ApplyMinMax=off  BusOutput=off  SignalInfo={'AMK_Reserve','12','4','LE','signed','Standard','0','1','0','0','15';'AMK_TargetVelocity','16','16','LE','signed','Standard','0','1','0','0','65535';'AMK_TorqueLimitNegativ','48','16','LE','signed','Standard','0','1','0','0','65535';'AMK_TorqueLimitPositiv','32','16','LE','signed','Standard','0','1','0','0','65535';'AMK_bEnable','10','1','LE','unsigned','Standard','0','1','0','0','1';'AMK_bErrorReset','11','1','LE','unsigned','Standard','0','1','0','0','1';'AMK_bInverterOn','8','1','LE','unsigned','Standard','0','1','0','0','1';'AMK_bReserve','0','8','LE','unsigned','Standard','0','1','0','0','255';'CAN_bdcon','9','1','LE','unsigned','Standard','0','1','0','0','1'}
      settings: SourceProductBaseCode=ME,XP,VN  DataFormat=CANdb specified signals
  CAN Pack2 : canmsglib/CAN Pack  CANdbFile=C:\Users\86155\Desktop\HRT2024\qkx\can\enable.dbc  MsgList=first_enable  MsgName=first_enable  MsgIDType=Standard (11-bit identifier)  MsgIdentifier=388  MsgLength=8  Remote=off  ApplyMinMax=off  BusOutput=off  SignalInfo={'AMK_Reserve','12','4','LE','signed','Standard','0','1','0','-8','7';'AMK_TargetVelocity','16','16','LE','signed','Standard','0','1','0','-32768','32767';'AMK_TorqueLimitNegativ','48','16','LE','signed','Standard','0','1','0','-32768','32767';'AMK_TorqueLimitPositiv','32','16','LE','signed','Standard','0','1','0','-32768','32767';'AMK_bEnable','10','1','LE','unsigned','Standard','0','1','0','0','1';'AMK_bErrorReset','11','1','LE','unsigned','Standard','0','1','0','0','1';'AMK_bInverterOn','8','1','LE','unsigned','Standard','0','1','0','0','1';'AMK_bReserve','0','8','LE','unsigned','Standard','0','1','0','0','255';'CAN_bdcon','9','1','LE','unsigned','Standard','0','1','0','0','1'}
      settings: SourceProductBaseCode=ME,XP,VN  DataFormat=CANdb specified signals
  CANPackMessage : ec5744lib/RapidECU_U4B/04CANCommunication/CANPackMessage  Commented=on  datalength=8  sampletime=-1
      settings: SourceProductName=ECUCoder for MPC5744
  CANPackMessage1 : ec5744lib/RapidECU_U4B/04CANCommunication/CANPackMessage  Commented=on  datalength=8  sampletime=-1
      settings: SourceProductName=ECUCoder for MPC5744
  CANPackMessage2 : ec5744lib/RapidECU_U4B/04CANCommunication/CANPackMessage  datalength=8  sampletime=-1
      settings: SourceProductName=ECUCoder for MPC5744
  CANTransmit : ec5744lib/RapidECU_U4B/04CANCommunication/CANTransmit  Commented=on  canmodule=0  canbuffer=10  canmessageid=hex2dec('189')  canmessagetype=Standard(11-bit ID)  datalength=8  sampletime=-1
      settings: SourceProductName=ECUCoder for MPC5744
  CANTransmit1 : ec5744lib/RapidECU_U4B/04CANCommunication/CANTransmit  canmodule=0  canbuffer=10  canmessageid=hex2dec('189')  canmessagetype=Standard(11-bit ID)  datalength=8  sampletime=-1
      settings: SourceProductName=ECUCoder for MPC5744
  Constant{,1..3,5,7..10,12,14,16..17,19} (14 alike) : Constant  Commented=on  Value=0  SampleTime=-1
  Constant{6,11,13,15} (4 alike) : Constant  Commented=on  SampleTime=-1
  Constant18 : Constant  Commented=on  Value=0
  Constant20 : Constant  Value=0  SampleTime=-1
  Constant4 : Constant  Value=0  SampleTime=-1
  Data Store Read1 : DataStoreRead  Commented=on  DataStoreName=zuohouvvv
  Data Store Read10 : DataStoreRead  DataStoreName=lcu_enable_189
  Data Store Read11 : DataStoreRead  Commented=on  DataStoreName=escmax
  Data Store Read12 : DataStoreRead  Commented=on  DataStoreName=V_workstation
  Data Store Read13 : DataStoreRead  DataStoreName=escmax
  Data Store Read14 : DataStoreRead  DataStoreName=V_workstation
  Data Store Read15 : DataStoreRead  DataStoreName=workstation_steering
  Data Store Read16 : DataStoreRead  DataStoreName=match_model
  Data Store Read17 : DataStoreRead  DataStoreName=huanting
  Data Store Read18 : DataStoreRead  DataStoreName=V_Kalman
  Data Store Read19 : DataStoreRead  DataStoreName=match_model
  Data Store Read2 : DataStoreRead  Commented=on  DataStoreName=lcu_enable_189
  Data Store Read20 : DataStoreRead  DataStoreName=yourenniuju
  Data Store Read21 : DataStoreRead  DataStoreName=oral_pressure_leftbehind
  Data Store Read3 : DataStoreRead  Commented=on  DataStoreName=lcu_enable_189_1
  Data Store Read4 : DataStoreRead  Commented=on  DataStoreName=huanting
  Data Store Read5 : DataStoreRead  Commented=on  DataStoreName=lcu_enable_189
  Data Store Read6 : DataStoreRead  DataStoreName=lcu_enable_189_1
  Data Store Read7 : DataStoreRead  Commented=on  DataStoreName=workstation_steering
  Data Store Read8 : DataStoreRead  DataStoreName=zuohouvvv
  Data Store Read9 : DataStoreRead  Commented=on  DataStoreName=match_model
  Data Store Write : DataStoreWrite  DataStoreName=energyr_zuohou
  Data Store Write1 : DataStoreWrite  DataStoreName=torque_zuohou
  Data Type Conversion : DataTypeConversion  Commented=on  OutDataTypeStr=uint8
  Data Type Conversion1 : DataTypeConversion  Commented=on  OutDataTypeStr=uint8
  Data Type Conversion2 : DataTypeConversion  OutDataTypeStr=uint8
  MATLAB Function : MATLAB Function  Commented=on  TreatAsAtomicUnit=on
  MATLAB Function1 : MATLAB Function  Commented=on  TreatAsAtomicUnit=on
  MATLAB Function2 : MATLAB Function  TreatAsAtomicUnit=on
  MATLAB Function3 : MATLAB Function  Commented=on  TreatAsAtomicUnit=on
  MATLAB Function4 : MATLAB Function  TreatAsAtomicUnit=on
  MATLAB Function5 : MATLAB Function  TreatAsAtomicUnit=on
  MATLAB Function6 : MATLAB Function  TreatAsAtomicUnit=on
  MATLAB Function7 : MATLAB Function  TreatAsAtomicUnit=on
  MeaModule : ec5744lib/RapidECU_U4B/07Calibration/MeaModule  Commented=on  signal=V189
      settings: SourceProductName=ECUCoder for MPC5744
  MeaModule1 : ec5744lib/RapidECU_U4B/07Calibration/MeaModule  Commented=on  signal=Vthird
      settings: SourceProductName=ECUCoder for MPC5744
  MeaModule2 : ec5744lib/RapidECU_U4B/07Calibration/MeaModule  signal=V189
      settings: SourceProductName=ECUCoder for MPC5744
  Switch{,1..3} (4 alike) : Switch  Commented=on  Criteria=u2 > Threshold
  Terminator : Terminator  Commented=on
  Terminator1 : Terminator
  无人制动标志位 : DataStoreRead  Commented=on  DataStoreName=wurenzhidongdeng
  无人制动标志位1 : DataStoreRead  DataStoreName=wurenzhidongdeng
  无人制动标志位3 : DataStoreRead  DataStoreName=wurenzhidongdeng
  油压传感器 : DataStoreRead  DataStoreName=ebszhidongyouya
  能量回收功率限制 : Subsystem
  wires:
  MeaModule2/1 -> Terminator1/1
  Data Type Conversion2/1 -> CANTransmit1/1
  CANPackMessage2/1 -> Data Type Conversion2/1
  CAN Pack2/1 -> CANPackMessage2/1
  CANTransmit1/1 -> MeaModule2/1
  MATLAB Function2/5(blnverteron) -> CAN Pack2/7
  Data Store Read10/1 -> MATLAB Function7/4(enable), MATLAB Function2/1("enable ")
  Data Store Read17/1 -> MATLAB Function4/4(huanting)
  Constant4/1 -> CAN Pack2/1
  Data Store Read16/1 -> MATLAB Function5/4(model)
  Data Store Read6/1 -> MATLAB Function7/5(enable_1), MATLAB Function2/2(enable_1)
  MATLAB Function2/4(errorreset) -> CAN Pack2/6
  MATLAB Function2/2(AMK_TorqueLimitPositive) -> CAN Pack2/4, Data Store Write1/1
  MATLAB Function2/6(CAN_dbcon) -> CAN Pack2/9
  MATLAB Function2/3(enable) -> CAN Pack2/5
  MATLAB Function2/1(TargetVelocity) -> CAN Pack2/2
  Constant20/1 -> CAN Pack2/8
  MATLAB Function4/1(y) -> MATLAB Function5/1(v)
  Data Store Read14/1 -> MATLAB Function4/1(u)
  Data Store Read15/1 -> MATLAB Function5/2(angle)
  无人制动标志位1/1 -> MATLAB Function4/3(zhidongebs)
  Data Store Read13/1 -> MATLAB Function4/2(zhidongesc)
  Data Store Read8/1 -> MATLAB Function5/3(vz)
  Data Store Read1/1 -> MATLAB Function3/3(vz)
  Data Store Read12/1 -> MATLAB Function/1(u)
  Data Store Read11/1 -> MATLAB Function/2(zhidongesc)
  无人制动标志位/1 -> MATLAB Function/3(zhidongebs)
  MATLAB Function1/1(T) -> Switch3/1
  Data Store Read9/1 -> MATLAB Function3/4(model)
  MATLAB Function/1(y) -> MATLAB Function3/1(v)
  MATLAB Function3/1(y) -> Switch2/3
  Data Store Read7/1 -> MATLAB Function3/2(angle)
  Data Store Read5/1 -> Switch3/2
  Switch3/1 -> CAN Pack1/4
  Constant19/1 -> Switch3/3
  MeaModule1/1 -> CAN Pack1/2
  Switch2/1 -> Switch1/1
  Constant18/1 -> Switch2/1
  Data Store Read4/1 -> Switch2/2
  Switch1/1 -> MeaModule1/1
  Data Store Read2/1 -> Switch1/2
  Constant17/1 -> Switch1/3
  Data Store Read3/1 -> Switch/2
  Switch/1 -> CANTransmit/1
  Data Type Conversion/1 -> Switch/3
  Data Type Conversion1/1 -> Switch/1
  Constant3/1 -> CAN Pack1/1
  Constant15/1 -> CAN Pack1/9
  CAN Pack1/1 -> CANPackMessage1/1
  CANPackMessage1/1 -> Data Type Conversion1/1
  Constant13/1 -> CAN Pack1/7
  Constant11/1 -> CAN Pack1/5
  Constant14/1 -> CAN Pack1/8
  Constant10/1 -> CAN Pack1/3
  Constant12/1 -> CAN Pack1/6
  MeaModule/1 -> Terminator/1
  CANTransmit/1 -> MeaModule/1
  Constant6/1 -> CAN Pack/6
  Constant2/1 -> CAN Pack/3
  Constant16/1 -> CAN Pack/4
  Constant1/1 -> CAN Pack/2
  Constant7/1 -> CAN Pack/7
  CAN Pack/1 -> CANPackMessage/1
  Constant9/1 -> CAN Pack/9
  CANPackMessage/1 -> Data Type Conversion/1
  Constant/1 -> CAN Pack/1
  Constant5/1 -> CAN Pack/5
  Constant8/1 -> CAN Pack/8
  Data Store Read19/1 -> MATLAB Function6/3(model)
  Data Store Read20/1 -> MATLAB Function6/2(youren)
  Data Store Read18/1 -> MATLAB Function5/7(vk), MATLAB Function6/1(v)
  MATLAB Function6/1(T) -> MATLAB Function2/3(T)
  MATLAB Function5/1(y) -> MATLAB Function2/4(v)
  无人制动标志位3/1 -> MATLAB Function5/5(zhidong)
  能量回收功率限制/1(T) -> MATLAB Function7/1(T)
  油压传感器/1 -> MATLAB Function7/3(youya)
  Data Store Read21/1 -> MATLAB Function5/6(T), MATLAB Function7/2(wurenyouya)
  MATLAB Function7/1(y) -> Data Store Write/1, CAN Pack2/3

== system control/Subsystem/Tx/Toworkstation/toworkstation/toworkstation ==
  CAN Pack : canmsglib/CAN Pack  CANdbFile=C:\Users\Liu keliang\Desktop\HRT2023\HRT23赛季刘科良\CANdbc\toworkstation.dbc  MsgList=(none)  MsgName=toworkstation  MsgIDType=Standard (11-bit identifier)  MsgIdentifier=562  MsgLength=8  Remote=off  ApplyMinMax=off  BusOutput=off  SignalInfo={'youhou','0','16','LE','signed','Standard','0','1','0','-Inf','Inf';'youqian','16','16','LE','signed','Standard','0','1','0','-Inf','Inf';'zuohou','32','16','LE','signed','Standard','0','1','0','-Inf','Inf';'zuoqian','48','16','LE','signed','Standard','0','1','0','-Inf','Inf'}
      settings: SourceProductBaseCode=ME,XP,VN  DataFormat=CANdb specified signals
  CAN Pack1 : canmsglib/CAN Pack  CANdbFile=C:\Users\Liu keliang\Desktop\HRT2023\HRT23赛季刘科良\CANdbc\ecuangle.dbc  MsgList=(none)  MsgName=New_Message_1  MsgIDType=Standard (11-bit identifier)  MsgIdentifier=563  MsgLength=2  Remote=off  ApplyMinMax=off  BusOutput=off  SignalInfo={'New_Signal_1','0','16','LE','signed','Standard','0','1','0','-1080','1080';'angelerror','16','8','LE','signed','Standard','0','1','0','-Inf','Inf'}
      settings: SourceProductBaseCode=ME,XP,VN  DataFormat=CANdb specified signals
  CANPackMessage : ec5744lib/RapidECU_U4B/04CANCommunication/CANPackMessage  datalength=8  sampletime=-1
      settings: SourceProductName=ECUCoder for MPC5744
  CANPackMessage1 : ec5744lib/RapidECU_U4B/04CANCommunication/CANPackMessage  datalength=2  sampletime=-1
      settings: SourceProductName=ECUCoder for MPC5744
  CANTransmit : ec5744lib/RapidECU_U4B/04CANCommunication/CANTransmit  canmodule=2  canbuffer=59  canmessageid=hex2dec('232')  canmessagetype=Standard(11-bit ID)  datalength=8  sampletime=-1
      settings: SourceProductName=ECUCoder for MPC5744
  CANTransmit1 : ec5744lib/RapidECU_U4B/04CANCommunication/CANTransmit  canmodule=2  canbuffer=63  canmessageid=hex2dec('233')  canmessagetype=Standard(11-bit ID)  datalength=2  sampletime=-1
      settings: SourceProductName=ECUCoder for MPC5744
  Data Store Read : DataStoreRead  DataStoreName=dianji_velcoity_zuoqian
  Data Store Read1 : DataStoreRead  DataStoreName=dianji_velcoity_youhou
  Data Store Read2 : DataStoreRead  DataStoreName=dianji_velcoity_youqian
  Data Store Read3 : DataStoreRead  DataStoreName=dianji_velcoity_zuohou
  Data Store Read4 : DataStoreRead  DataStoreName=zhuanjiao_1
  Data Store Read5 : DataStoreRead  DataStoreName=steere
  Data Type Conversion : DataTypeConversion  OutDataTypeStr=uint8
  Data Type Conversion1 : DataTypeConversion  OutDataTypeStr=uint8
  Gain{,1..3} (4 alike) : Gain  Gain=594.06
  MeaModule : ec5744lib/RapidECU_U4B/07Calibration/MeaModule  signal=T232
      settings: SourceProductName=ECUCoder for MPC5744
  MeaModule1 : ec5744lib/RapidECU_U4B/07Calibration/MeaModule  signal=T233
      settings: SourceProductName=ECUCoder for MPC5744
  Terminator : Terminator
  Terminator1 : Terminator
  wires:
  CANPackMessage/1 -> Data Type Conversion/1
  CAN Pack/1 -> CANPackMessage/1
  CANTransmit/1 -> MeaModule/1
  MeaModule/1 -> Terminator/1
  Data Type Conversion/1 -> CANTransmit/1
  Data Store Read/1 -> Gain3/1
  Data Store Read1/1 -> Gain/1
  Data Store Read2/1 -> Gain1/1
  Data Store Read3/1 -> Gain2/1
  CANTransmit1/1 -> MeaModule1/1
  MeaModule1/1 -> Terminator1/1
  CANPackMessage1/1 -> Data Type Conversion1/1
  CAN Pack1/1 -> CANPackMessage1/1
  Data Type Conversion1/1 -> CANTransmit1/1
  Data Store Read4/1 -> CAN Pack1/1
  Data Store Read5/1 -> CAN Pack1/2
  Gain/1 -> CAN Pack/1
  Gain1/1 -> CAN Pack/2
  Gain2/1 -> CAN Pack/3
  Gain3/1 -> CAN Pack/4

== system control/Subsystem/Tx/Toworkstation/转向/Subsystem ==
  Enable : EnablePort
  MATLAB Function : MATLAB Function  TreatAsAtomicUnit=on
  MATLAB Function1 : MATLAB Function  TreatAsAtomicUnit=on
  Subsystem : Subsystem
  Subsystem1 : Subsystem
  wires:
  MATLAB Function/1(biaozhi1) -> Subsystem/Enable
  MATLAB Function1/2(y2) -> Subsystem1/2(y2)
  MATLAB Function1/1(y1) -> Subsystem1/1(y1)
  MATLAB Function1/3(biaozhi2) -> Subsystem1/Enable
